simulink model "LQR_single_brady"  (R2016a)
settings: Solver=FixedStepAuto  SolverMode=SingleTasking  StartTime=0.0  StopTime=24.9  FixedStep=0.0001  RelTol=1e-3
values from neighbouring files (symbols this model uses):
  Cf = 30989    [LQR_Setup.m]
  Cr = 50154    [LQR_Setup.m]
  Iz = 111.8    [LQR_Setup.m]
  K1l = K(1,1)    [LQR_Setup.m]
  K2l = K(1,2)    [LQR_Setup.m]
  K3l = K(1,3)    [LQR_Setup.m]
  lf = 0.783    [LQR_Setup.m]
  lr = 0.752    [LQR_Setup.m]
  m = 245    [LQR_Setup.m]
undefined symbols (not defined in the file or in its folder): DiscIntNeverNeededParam
settings Model: Creator=Johan PC  LastModifiedBy=Johan PC
settings DebuggingCC: SFUnexpectedBacktrackingDiag=error  SFNoUnconditionalDefaultTransitionDiag=error
settings SFSimCC: SimUseLocalCustomCode=on
settings RTWCC: RTWUseLocalCustomCode=on
settings GRTTargetCC: TargetLangStandard=C99 (ISO)  GeneratePreprocessorConditionals=Use local settings
settings ConfigComp: CovMetricSettings=dwe  CovHtmlReporting=off  CovSaveCumulativeToWorkspaceVar=off  CovSaveSingleToWorkspaceVar=off  CovExternalEMLEnable=on

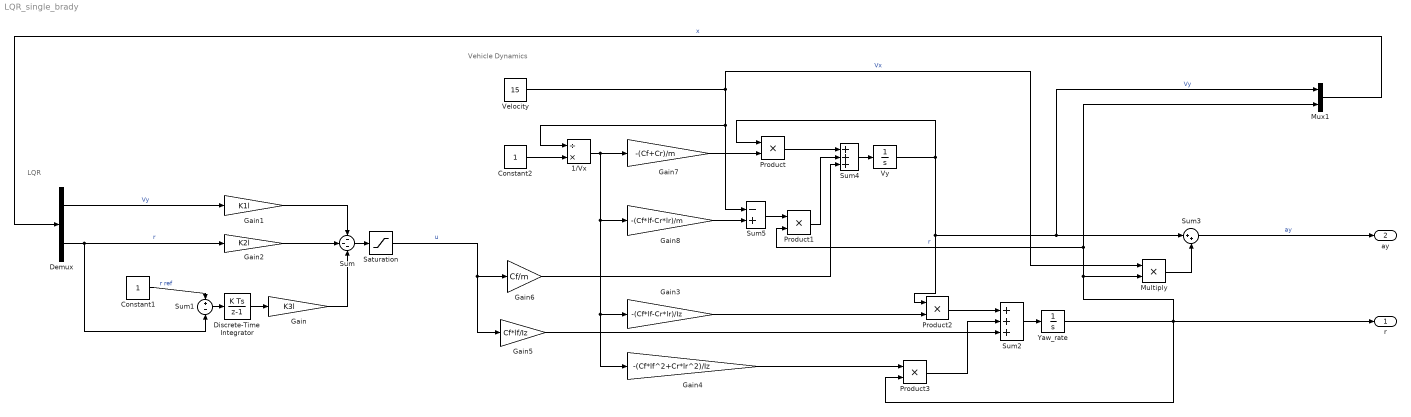
== system LQR_single_brady ==
  note: Vehicle Dynamics
  note: LQR
  1/Vx : Product  Inputs=/*
  Constant1 : Constant
  Constant2 : Constant
  Demux : Demux  Outputs=2
  Discrete-Time Integrator : DiscreteIntegrator  InitialConditionSetting=State (most efficient)  SampleTime=0.001  ICPrevOutput=DiscIntNeverNeededParam  ICPrevScaledInput=DiscIntNeverNeededParam
  Gain : Gain  Gain=K3l
  Gain1 : Gain  Gain=K1l
  Gain2 : Gain  Gain=K2l
  Gain3 : Gain  Gain=-(Cf*lf-Cr*lr)/Iz
  Gain4 : Gain  Gain=-(Cf*lf^2+Cr*lr^2)/Iz
  Gain5 : Gain  Gain=Cf*lf/Iz
  Gain6 : Gain  Gain=Cf/m
  Gain7 : Gain  Gain=-(Cf+Cr)/m
  Gain8 : Gain  Gain=-(Cf*lf-Cr*lr)/m
  Multiply : Product
  Mux1 : Mux  Inputs=2
  Product{,1..3} (4 alike) : Product
  Saturation : Saturate  UpperLimit=0.45  LowerLimit=-0.45
  Sum : Sum  Inputs=---
  Sum1 : Sum  Inputs=+-
  Sum2 : Sum  Inputs=+++
  Sum3 : Sum  Inputs=|++
  Sum4 : Sum  Inputs=+++
  Sum5 : Sum  Inputs=-+
  Velocity : Constant  Value=15
  Vy : Integrator
  "Yaw_rate " : Integrator
  r : Outport
  ay : Outport  Port=2
  wires:
  Constant1/1 -> Sum1/1  "r ref"
  Sum1/1 -> Discrete-Time Integrator/1
  Sum/1 -> Saturation/1
  Gain2/1 -> Sum/2
  Gain1/1 -> Sum/1
  Demux/2 -> Sum1/2, Gain2/1  "r"
  Demux/1 -> Gain1/1  "Vy"
  Mux1/1 -> Demux/1  "x"
  Gain/1 -> Sum/3
  Discrete-Time Integrator/1 -> Gain/1
  Sum3/1 -> ay/1  "ay"
  Multiply/1 -> Sum3/2
  Product1/1 -> Sum4/2
  Velocity/1 -> Multiply/1, 1/Vx/1, Sum5/1  "Vx"
  Sum4/1 -> Vy/1
  Vy/1 -> Mux1/1, Sum3/1, Product2/1, Product/1  "Vy"
  Product/1 -> Sum4/1
  Gain7/1 -> Product/2
  Saturation/1 -> Gain6/1, Gain5/1  "u"
  Gain6/1 -> Sum4/3
  "Yaw_rate "/1 -> r/1, Mux1/2, Product1/2, Multiply/2, Product3/2  "r"
  Sum5/1 -> Product1/1
  Gain5/1 -> Sum2/3
  Product3/1 -> Sum2/2
  Product2/1 -> Sum2/1
  1/Vx/1 -> Gain4/1, Gain3/1, Gain8/1, Gain7/1
  Gain3/1 -> Product2/2
  Constant2/1 -> 1/Vx/2
  Gain4/1 -> Product3/1
  Gain8/1 -> Sum5/2
  Sum2/1 -> "Yaw_rate "/1
